simulink model "main_Sim"  (R2016a)
settings: Solver=VariableStepAuto  StartTime=0.0  StopTime=10.0  RelTol=1e-3
settings Model: Creator=SRQ  LastModifiedBy=SRQ
settings DataIOCC: LimitDataPoints=on
settings DebuggingCC: AllowSymbolicDim=off
settings ModelReferenceCC: PropagateSignalLabelsOutOfModel=off
settings GRTTargetCC: GeneratePreprocessorConditionals=Use local settings

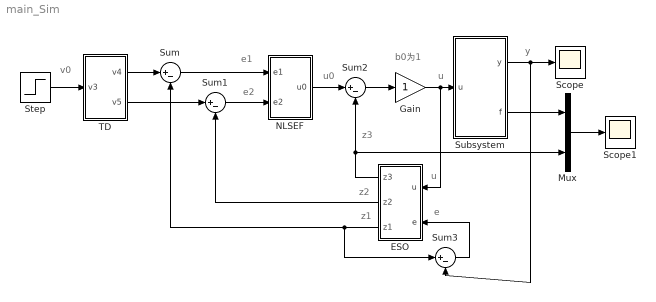
== system main_Sim ==
  note: e
  note: u
  note: z1
  note: z2
  note: z3
  note: u
  note: y
  note: b0为1
  note: u0
  note: e2
  note: e1
  note: v0
  ESO : Subsystem  mask(ESO){h=0.01, beta_01=100, beta_02=300, beta_03=1000, b0=1}
      mask help: 这一部分（扩张状态观测器）的作用是得到系统状态变量的估计值及扩张状态的实时作用量。
      mask Display: disp('ESO');
  Gain : Gain
  Mux : Mux  Inputs=2
  NLSEF : Subsystem  mask(NLSEF){c=0.3, r=5, h1=0.03}
      mask help: 非线性状态误差反馈律是把跟踪微分器产生的跟踪信号和微分信号与扩张状态观测器得到的系统的状态估计通过非线性函数进行适当组合，作为被控对象的控制量。
      mask Display: disp('NLSEF');
  Scope : Scope
  Scope1 : Scope
  Step : Step  Time=0  SampleTime=0
  Subsystem : Subsystem
      mask Display: disp('PLANT');
  Sum{,1..3} (4 alike) : Sum  Inputs=|+-
  TD : Subsystem  mask(TD){r0=2.0, h=0.01}
      mask help: 跟踪微分器为系统输入安排过渡过程，得到光滑的输入信号以及输入信号的微分信号。
      mask Display: disp('TD');
  wires:
  Step/1 -> TD/1(v3)
  TD/1(v4) -> Sum/1
  TD/2(v5) -> Sum1/1
  Sum/1 -> NLSEF/1(e1)
  Sum1/1 -> NLSEF/2(e2)
  NLSEF/1(u0) -> Sum2/1
  Sum2/1 -> Gain/1
  Gain/1 -> ESO/1(u), Subsystem/1(u)
  Subsystem/1(y) -> Sum3/2, Scope/1
  Subsystem/2(f) -> Mux/1
  ESO/1(z3) -> Mux/2, Sum2/2
  ESO/2(z2) -> Sum1/2
  ESO/3(z1) -> Sum3/1, Sum/2
  Sum3/1 -> ESO/2(e)
  Mux/1 -> Scope1/1

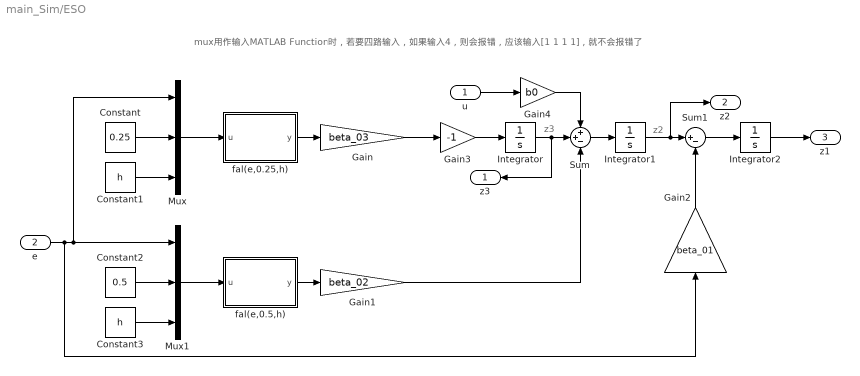
== system main_Sim/ESO ==
  note: z2
  note: z3
  note: mux用作输入MATLAB Function时，若要四路输入，如果输入4，则会报错，应该输入[1 1 1 1]，就不会报错了
  u : Inport
  e : Inport  Port=2
  Constant : Constant  Value=0.25
  Constant1 : Constant  Value=h
  Constant2 : Constant  Value=0.5
  Constant3 : Constant  Value=h
  Gain : Gain  Gain=beta_03
  Gain1 : Gain  Gain=beta_02
  Gain2 : Gain  Gain=beta_01
  Gain3 : Gain  Gain=-1
  Gain4 : Gain  Gain=b0
  Integrator : Integrator
  Integrator1 : Integrator
  Integrator2 : Integrator
  Mux : Mux  Inputs=[1 1 1]
  Mux1 : Mux  Inputs=[1 1 1]
  Sum : Sum  Inputs=++-
  Sum1 : Sum  Inputs=|+-
  fal(e,0.25,h) : MATLAB Function  TreatAsAtomicUnit=on
  fal(e,0.5,h) : MATLAB Function  TreatAsAtomicUnit=on
  z3 : Outport
  z2 : Outport  Port=2
  z1 : Outport  Port=3
  wires:
  Mux1/1 -> fal(e,0.5,h)/1(u)
  Mux/1 -> fal(e,0.25,h)/1(u)
  e/1 -> Gain2/1, Mux/1, Mux1/1
  Constant1/1 -> Mux/3
  Sum/1 -> Integrator1/1
  Gain2/1 -> Sum1/2
  Constant2/1 -> Mux1/2
  Gain4/1 -> Sum/1
  Integrator/1 -> z3/1, Sum/2
  fal(e,0.25,h)/1(y) -> Gain/1
  u/1 -> Gain4/1
  Gain1/1 -> Sum/3
  Constant3/1 -> Mux1/3
  Constant/1 -> Mux/2
  Integrator1/1 -> z2/1, Sum1/1
  Gain/1 -> Gain3/1
  Gain3/1 -> Integrator/1
  Sum1/1 -> Integrator2/1
  fal(e,0.5,h)/1(y) -> Gain1/1
  Integrator2/1 -> z1/1

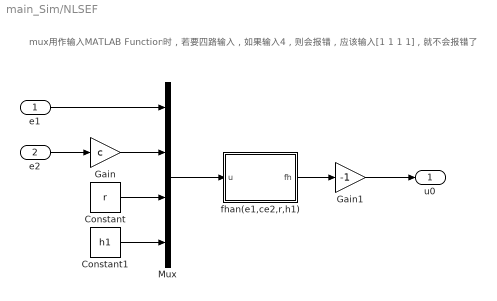
== system main_Sim/NLSEF ==
  note: mux用作输入MATLAB Function时，若要四路输入，如果输入4，则会报错，应该输入[1 1 1 1]，就不会报错了
  e1 : Inport
  e2 : Inport  Port=2
  Constant : Constant  Value=r
  Constant1 : Constant  Value=h1
  Gain : Gain  Gain=c
  Gain1 : Gain  Gain=-1
  Mux : Mux  Inputs=[1 1 1 1]
  fhan(e1,ce2,r,h1) : MATLAB Function  TreatAsAtomicUnit=on
  u0 : Outport
  wires:
  Mux/1 -> fhan(e1,ce2,r,h1)/1(u)
  Constant/1 -> Mux/3
  e2/1 -> Gain/1
  e1/1 -> Mux/1
  Constant1/1 -> Mux/4
  fhan(e1,ce2,r,h1)/1(fh) -> Gain1/1
  Gain1/1 -> u0/1
  Gain/1 -> Mux/2

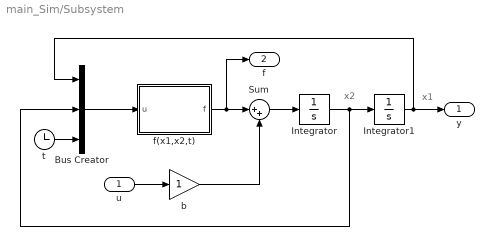
== system main_Sim/Subsystem ==
  note: x1
  note: x2
  u : Inport
  Bus Creator : BusCreator  Inputs=3
  Integrator : Integrator
  Integrator1 : Integrator
  Sum : Sum  Inputs=|++
  b : Gain
  f(x1,x2,t) : MATLAB Function  TreatAsAtomicUnit=on
  t : Clock
  y : Outport
  f : Outport  Port=2
  wires:
  t/1 -> Bus Creator/3
  u/1 -> b/1
  Bus Creator/1 -> f(x1,x2,t)/1(u)
  f(x1,x2,t)/1(f) -> f/1, Sum/1
  b/1 -> Sum/2
  Sum/1 -> Integrator/1
  Integrator/1 -> Bus Creator/2, Integrator1/1
  Integrator1/1 -> Bus Creator/1, y/1

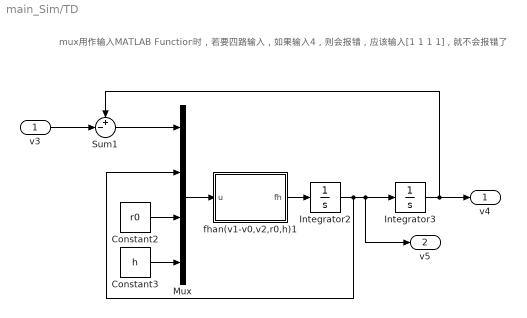
== system main_Sim/TD ==
  note: mux用作输入MATLAB Function时，若要四路输入，如果输入4，则会报错，应该输入[1 1 1 1]，就不会报错了
  v3 : Inport
  Constant2 : Constant  Value=r0
  Constant3 : Constant  Value=h
  Integrator2 : Integrator
  Integrator3 : Integrator
  Mux : Mux  Inputs=[1 1 1 1]
  Sum1 : Sum  Inputs=+-|
  fhan(v1-v0,v2,r0,h)1 : MATLAB Function  TreatAsAtomicUnit=on
  v4 : Outport
  v5 : Outport  Port=2
  wires:
  Constant2/1 -> Mux/3
  Mux/1 -> fhan(v1-v0,v2,r0,h)1/1(u)
  v3/1 -> Sum1/2
  fhan(v1-v0,v2,r0,h)1/1(fh) -> Integrator2/1
  Integrator2/1 -> v5/1, Integrator3/1, Mux/2
  Sum1/1 -> Mux/1
  Constant3/1 -> Mux/4
  Integrator3/1 -> v4/1, Sum1/1

== matlab function main_Sim/NLSEF/fhan(e1,ce2,r,h1) ==
  data: u input; fh output
function fh = fcn(u)
%#codegen 非线性函数fhan(x1,x2,r,h)
x1 = u(1);
x2 = u(2);
r = u(3);
h = u(4);

d = r * h * h;
a0 = h * x2;
y = x1 + a0;
a1 = sqrt(d * (d + 8 * abs(y)));
a2 = a0 + sign(y) * (a1 - d) / 2;
sy = (sign(y + d) - sign(y - d)) / 2;
a = (a0 + y - a2) * sy + a2;
sa = (sign(a + d) - sign(a - d)) / 2;

fh = -r * (a / d - sign(a)) * sa - r * sign(a);

== matlab function main_Sim/Subsystem/f(x1,x2,t) ==
  data: u input; f output
function f = fcn(u)
%#codegen
x1 = u(1);
x2 = u(2);
t = u(3);

gamma1 = 1.0;
gamma2 = 1.0;
omega1 = 0.6;
omega2 = 0.7;
omega = 1.0;

f = gamma1 * cos(omega1 * t) * x1 + gamma2 * cos(omega2 * t) * x2 + 0.5 * sign(sin(omega * t));

== matlab function main_Sim/ESO/fal(e,0.25,h) ==
  data: u input; y output
function y = fcn(u)
%#codegen 非线性函数fal(x,α,d)
x = u(1);
alpha = u(2);
d = u(3);

if abs(x) <= d
    y = x / (d ^ (1 - alpha));
else 
    y = abs(x) ^ alpha * sign(x);
end

== matlab function main_Sim/ESO/fal(e,0.5,h) ==
  data: u input; y output
function y = fcn(u)
%#codegen 非线性函数fal(x,α,d)
x = u(1);
alpha = u(2);
d = u(3);

if abs(x) <= d
    y = x / (d ^ (1 - alpha));
else 
    y = abs(x) ^ alpha * sign(x);
end

== matlab function main_Sim/TD/fhan(v1-v0,v2,r0,h)1 ==
  data: u input; fh output
function fh = fcn(u)
%#codegen 非线性函数fhan(x1,x2,r,h)
x1 = u(1);
x2 = u(2);
r = u(3);
h = u(4);

d = r * h * h;
a0 = h * x2;
y = x1 + a0;
a1 = sqrt(d * (d + 8 * abs(y)));
a2 = a0 + sign(y) * (a1 - d) / 2;
sy = (sign(y + d) - sign(y - d)) / 2;
a = (a0 + y - a2) * sy + a2;
sa = (sign(a + d) - sign(a - d)) / 2;

fh = -r * (a / d - sign(a)) * sa - r * sign(a);
